simulink model "BLDC"  (R2016b)
settings: Solver=VariableStepAuto  StartTime=0.0  StopTime=3  RelTol=1e-3
libraries: powerlib x9
settings Model: Creator=WANGSP1  LastModifiedBy=USER
settings SolverCC: ZeroCrossAlgorithm=Adaptive

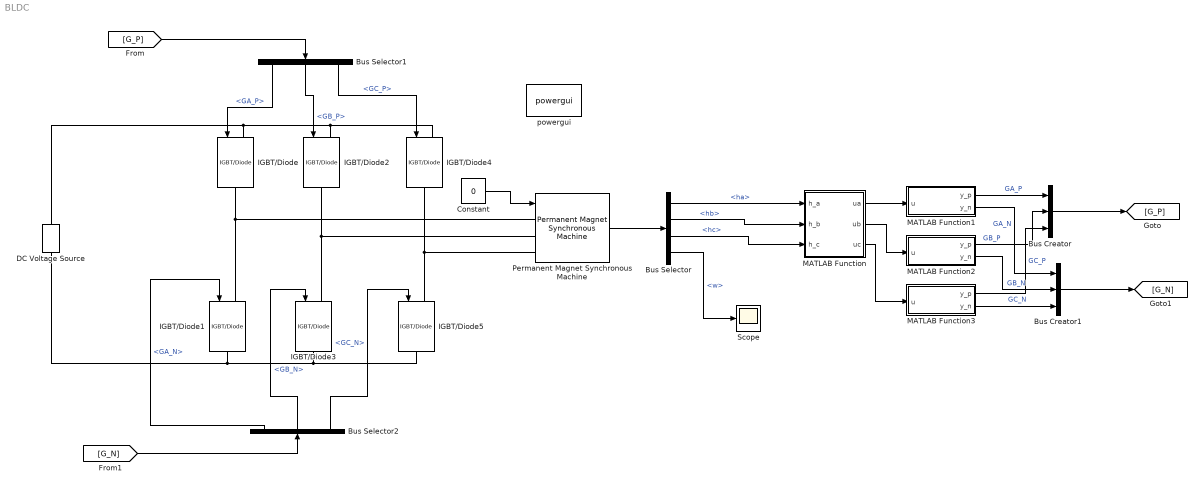
== system BLDC ==
  Bus Creator : BusCreator  Inputs=3
  Bus Creator1 : BusCreator  Inputs=3
  Bus Selector : BusSelector  OutputSignals=ha,hb,hc,w
  Bus Selector1 : BusSelector  OutputSignals=GA_P,GB_P,GC_P
  Bus Selector2 : BusSelector  OutputSignals=GA_N,GB_N,GC_N
  Constant : Constant  Value=0
  DC Voltage Source : powerlib/Electrical Sources/DC Voltage Source  Amplitude=100  Measurements=None
  IGBT/Diode{,1..5} (6 alike) : powerlib/Power Electronics/IGBT//Diode  Ron=1e-3  Rs=1e5  Cs=inf  Measurements=off
  MATLAB Function : MATLAB Function  TreatAsAtomicUnit=on
  MATLAB Function1 : MATLAB Function  TreatAsAtomicUnit=on
  MATLAB Function2 : MATLAB Function  TreatAsAtomicUnit=on
  MATLAB Function3 : MATLAB Function  TreatAsAtomicUnit=on
  Permanent Magnet Synchronous Machine : powerlib/Machines/Permanent Magnet Synchronous Machine  NbPhases=3  FluxDistribution=Trapezoidal  RotorType=Round  MechanicalLoad=Torque Tm  PresetModel="01:  0.8 Nm 300 Vdc 3000 RPM - 0.8 Nm"  ShowDetailedParameters=on  MeasurementBus=on  Resistance=18.7  Inductance=8.5e-3  dqInductances=[8.5e-3,8.5e-3]  La=0.02682  MachineConstant=Torque Constant (N.m / A_peak)  Flux=0.13181  VoltageCst=55.2135  TorqueCst=0.52725  Flat=120  Mechanical=[2.26e-03 1.349e-05 2 0]  PolePairs=2  InitialConditions=[0,0, 0,0]  InitialConditions5ph=[0 0 0 0 0 0]  TsPowergui=0  TsBlock=-1  RefAngle=Aligned with phase A axis (original Park)
  Scope : Scope
  powergui : powerlib/powergui  Priority=1  SimulationMode=Continuous  SolverType=Tustin/Backward Euler (TBE)  SampleTime=50e-6  frequency=60  SPID=off  DisableSnubberDevices=off  DisableRonSwitches=off  DisableVfSwitches=off  SwTol=0  DisplayEquations=off  Interpol=off  ExternalGateDelay=off  methode=off  Ts=10  FunctionMessages=off  echomessages=off  HookPort=off  EnableUseOfTLC=off  x0status=blocks  frequencyindice=0  Pbase=100e6  ErrMax=1e-4  Iterations=50  UnitsV=kV  UnitsW=MW  buscounter=0  RestoreLinks=warning  ResistiveCurrentMeasurement=off  Frange=[0:2:500]  Ylog=off  Xlog=on  ShowGrid=off  save=off  variable=ZData  structure=0  ZoomFFT=off  StartTime=0.0  cycles=1  DisplayStyle=1  fundamental=60  FreqAxis=off  MaxFrequency=1000  frequencyindicesteady=1  RmsSteady=1  display=off
  wires:
  Permanent Magnet Synchronous Machine/1 -> Bus Selector/1
  Bus Selector/1 -> MATLAB Function/1(h_a)  "<ha>"
  Bus Selector/2 -> MATLAB Function/2(h_b)  "<hb>"
  Bus Selector/3 -> MATLAB Function/3(h_c)  "<hc>"
  MATLAB Function/1(ua) -> MATLAB Function1/1(u)
  MATLAB Function/2(ub) -> MATLAB Function2/1(u)
  MATLAB Function/3(uc) -> MATLAB Function3/1(u)
  MATLAB Function1/1(y_p) -> Bus Creator/1  "GA_P"
  MATLAB Function2/1(y_p) -> Bus Creator/2  "GB_P"
  MATLAB Function3/1(y_p) -> Bus Creator/3  "GC_P"
  Bus Creator/1 -> [G_P]
  Bus Creator1/1 -> [G_N]
  MATLAB Function3/2(y_n) -> Bus Creator1/3  "GC_N"
  MATLAB Function1/2(y_n) -> Bus Creator1/1  "GA_N"
  MATLAB Function2/2(y_n) -> Bus Creator1/2  "GB_N"
  [G_P] -> Bus Selector1/1
  Bus Selector1/2 -> IGBT/Diode2/1  "<GB_P>"
  [G_N] -> Bus Selector2/1
  Bus Selector2/1 -> IGBT/Diode1/1  "<GA_N>"
  Bus Selector2/2 -> IGBT/Diode3/1  "<GB_N>"
  Bus Selector2/3 -> IGBT/Diode5/1  "<GC_N>"
  Bus Selector/4 -> Scope/1  "<w>"
  Constant/1 -> Permanent Magnet Synchronous Machine/1
  Bus Selector1/1 -> IGBT/Diode/1  "<GA_P>"
  Bus Selector1/3 -> IGBT/Diode4/1  "<GC_P>"
  connections:
  IGBT/Diode1/LConn1 -- Permanent Magnet Synchronous Machine/LConn1 -- IGBT/Diode/RConn1
  IGBT/Diode3/LConn1 -- Permanent Magnet Synchronous Machine/LConn2 -- IGBT/Diode2/RConn1
  IGBT/Diode5/LConn1 -- Permanent Magnet Synchronous Machine/LConn3 -- IGBT/Diode4/RConn1
  IGBT/Diode/LConn1 -- DC Voltage Source/RConn1 -- IGBT/Diode4/LConn1 -- IGBT/Diode2/LConn1
  IGBT/Diode1/RConn1 -- DC Voltage Source/LConn1 -- IGBT/Diode5/RConn1 -- IGBT/Diode3/RConn1

== matlab function BLDC/MATLAB Function1 ==
  data: u input; y_p output; y_n output
function [y_p,y_n] = fcn(u)
if(u==1)
    y_p=1;y_n=0;
else
    if(u==-1)
        y_p=0;y_n=1;
    else
        y_p=0;y_n=0;
    end
end

== matlab function BLDC/MATLAB Function ==
  data: h_a input; ua output; h_b input; h_c input; ub output; uc output
function [ua,ub,uc] = fcn(h_a,h_b,h_c)
tmp=h_a*4+h_b*2+h_c;
switch(tmp)
    case 1
        ua=1;ub=0;uc=-1;
    case 0
        ua=1;ub=-1;uc=0;
    case 4
        ua=0;ub=-1;uc=1;
    case 6
        ua=-1;ub=0;uc=1;
    case 7
        ua=-1;ub=1;uc=0;
    case 3
        ua=0;ub=1;uc=-1;
    otherwise
        ua=0;ub=0;uc=0;      
end

== matlab function BLDC/MATLAB Function2 ==
  data: u input; y_p output; y_n output
function [y_p,y_n] = fcn(u)
if(u==1)
    y_p=1;y_n=0;
else
    if(u==-1)
        y_p=0;y_n=1;
    else
        y_p=0;y_n=0;
    end
end

== matlab function BLDC/MATLAB Function3 ==
  data: u input; y_p output; y_n output
function [y_p,y_n] = fcn(u)
if(u==1)
    y_p=1;y_n=0;
else
    if(u==-1)
        y_p=0;y_n=1;
    else
        y_p=0;y_n=0;
    end
end
